simulink model "velo_test"  (R2025b)
settings: Solver=VariableStepAuto  StartTime=0.0  StopTime=10.0  RelTol=1e-3
libraries: arduino_io_lib x5
settings Model: Creator=nttha  LastModifiedBy=nttha

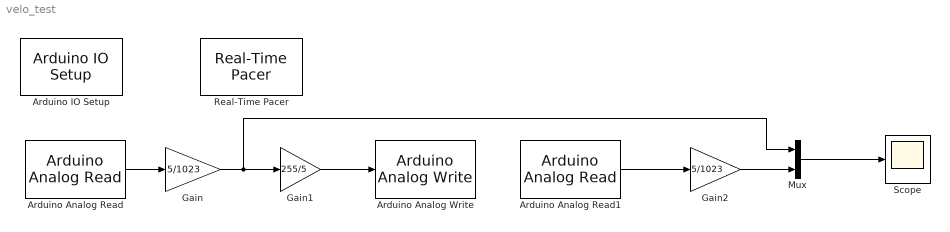
== system velo_test ==
  Arduino Analog Read : arduino_io_lib/Arduino Analog Read  arduinoVar=Temporary arduino variable: Arduino1  arduinoPin=1  T=0.02
      settings: SourceProductName=Arduino IO Library
  Arduino Analog Read1 : arduino_io_lib/Arduino Analog Read  arduinoVar=Temporary arduino variable: Arduino1  arduinoPin=0  T=0.02
      settings: SourceProductName=Arduino IO Library
  Arduino Analog Write : arduino_io_lib/Arduino Analog Write  arduinoVar=Temporary arduino variable: Arduino1  arduinoPin=3  T=0.02
      settings: SourceProductName=Arduino IO Library
  Arduino IO Setup : arduino_io_lib/Arduino IO Setup  Priority=3  arduinoVar=Temporary arduino variable: Arduino1  workspaceVarName=a  comPort=COM3
      settings: SourceProductName=Arduino IO Library
  Gain : Gain  Gain=5/1023
  Gain1 : Gain  Gain=255/5
  Gain2 : Gain  Gain=5/1023
  Mux : Mux  Inputs=2
  Real-Time Pacer : arduino_io_lib/Real-Time Pacer  simTimePerRealTime=1
      settings: SourceProductName=Arduino IO Library
  Scope : Scope
      settings: ActiveDisplayYMinimum=-0.47715053763440851  ActiveDisplayYMaximum=4.2943548387096779
  wires:
  Arduino Analog Read/1 -> Gain/1
  Gain/1 -> Mux/1, Gain1/1
  Gain1/1 -> Arduino Analog Write/1
  Arduino Analog Read1/1 -> Gain2/1
  Gain2/1 -> Mux/2
  Mux/1 -> Scope/1
